simulink model "VehicleControl"  (R2021b)
settings: Solver=FixedStepDiscrete  StartTime=0.0  StopTime=10.0  FixedStep=0.01  RelTol=1e-3
undefined symbols (not defined in the file): DiscIntNeverNeededParam
libraries: simulink x9, simulink_extras x1
settings Model: Creator=Admin  LastModifiedBy=Admin
settings OptimizationCC: DefaultParameterBehavior=Inlined  UseDivisionForNetSlopeComputation=on  GainParamInheritBuiltInType=on  UseFloatMulNetSlope=on  InlineInvariantSignals=on  PassReuseOutputArgsAs=Individual arguments  ZeroExternalMemoryAtStartup=off  ZeroInternalMemoryAtStartup=off  NoFixptDivByZeroProtection=on  EfficientFloat2IntCast=on  LifeSpan=1  OptimizeBlockOrder=speed  DifferentSizesBufferReuse=on  EfficientTunableParamExpr=on
settings DebuggingCC: ParameterTunabilityLossMsg=error
settings HardwareCC: ProdLongLongMode=on
settings ModelReferenceCC: EnableRefExpFcnMdlSchedulingChecks=off
settings SFSimCC: MATLABDynamicMemAlloc=off
settings RTWCC: Description=Embedded Coder  SystemTargetFile=ert.tlc  PackageName=RemoteControllerCodeGen  TemplateMakefile=ert_default_tmf
settings CodeAppCC: ForceParamTrailComments=on  IgnoreCustomStorageClasses=off  OperatorAnnotations=on  SimulinkDataObjDesc=on  SFDataObjDesc=on  CustomSymbolStrGlobalVar=rt$N$M  CustomSymbolStrType=$N$M  CustomSymbolStrFcn=$N$M$F  CustomSymbolStrMacro=$N$M  InsertBlockDesc=on
settings ERTTargetCC: TargetLangStandard=C99 (ISO)  GenerateSampleERTMain=on  IncludeMdlTerminateFcn=off  CombineSignalStateStructs=on  SupportAbsoluteTime=off  SupportComplex=off  SupportNonInlinedSFcns=on  InlinedParameterPlacement=NonHierarchical  ERTCustomFileTemplate=example_file_process.tlc  ERTFilePackagingFormat=CompactWithDataFile

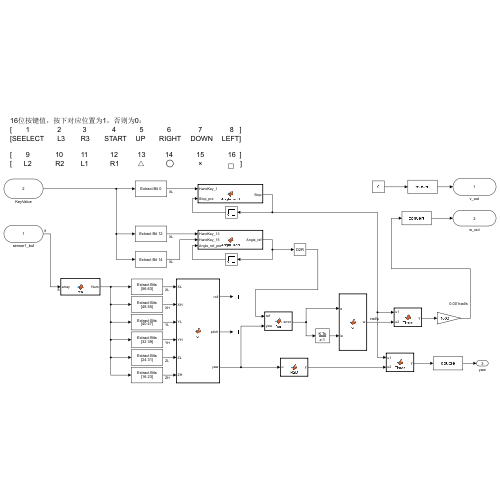
[thumbnail: Simulink's stored preview of the top-level diagram]
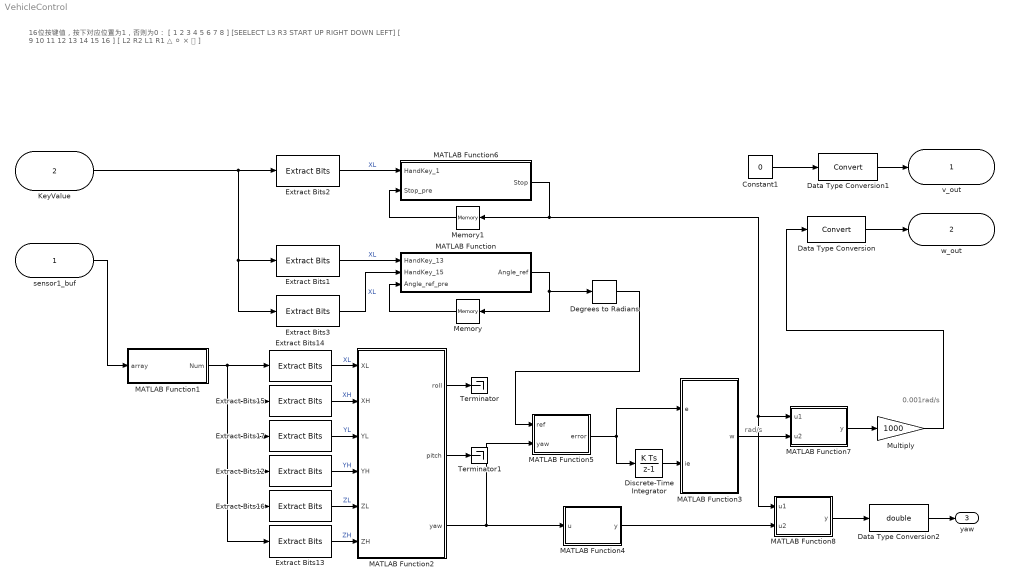
== system VehicleControl ==
  note: 16位按键值，按下对应位置为1，否则为0：
      | [ 1 2 3 4 5 6 7 8 ]
      | [SEELECT L3 R3 START UP RIGHT DOWN LEFT]
      |
      | [ 9 10 11 12 13 14 15 16 ]
      | [ L2 R2 L1 R1 △ ⚪ × ⃞ ]
  note: 0.001rad/s
  note: rad/s
  sensor1_buf : Inport  OutDataTypeStr=int8  PortDimensions=8
  KeyValue : Inport  Port=2  OutDataTypeStr=uint16  PortDimensions=1
  Constant1 : Constant  Value=0  OutDataTypeStr=uint8  SampleTime=-1
  Data Type Conversion : DataTypeConversion
  Data Type Conversion1 : DataTypeConversion
  Data Type Conversion2 : DataTypeConversion  OutDataTypeStr=double
  Degrees to Radians : simulink_extras/Transformations/Degrees to Radians
  Discrete-Time Integrator : DiscreteIntegrator  SampleTime=-1  ICPrevOutput=DiscIntNeverNeededParam  ICPrevScaledInput=DiscIntNeverNeededParam
  Extract Bits1 : simulink/Logic and Bit Operations/Extract Bits  bitsToExtract=Range of bits  numBits=8  bitIdxRange=[12]  outScalingMode=Treat bit field as an integer
  Extract Bits12 : simulink/Logic and Bit Operations/Extract Bits  bitsToExtract=Range of bits  numBits=8  bitIdxRange=[32 39]  outScalingMode=Treat bit field as an integer
  Extract Bits13 : simulink/Logic and Bit Operations/Extract Bits  bitsToExtract=Range of bits  numBits=8  bitIdxRange=[16 23]  outScalingMode=Treat bit field as an integer
  Extract Bits14 : simulink/Logic and Bit Operations/Extract Bits  bitsToExtract=Range of bits  numBits=8  bitIdxRange=[56 63]  outScalingMode=Treat bit field as an integer
  Extract Bits15 : simulink/Logic and Bit Operations/Extract Bits  bitsToExtract=Range of bits  numBits=8  bitIdxRange=[48 55]  outScalingMode=Treat bit field as an integer
  Extract Bits16 : simulink/Logic and Bit Operations/Extract Bits  bitsToExtract=Range of bits  numBits=8  bitIdxRange=[24 31]  outScalingMode=Treat bit field as an integer
  Extract Bits17 : simulink/Logic and Bit Operations/Extract Bits  bitsToExtract=Range of bits  numBits=8  bitIdxRange=[40 47]  outScalingMode=Treat bit field as an integer
  Extract Bits2 : simulink/Logic and Bit Operations/Extract Bits  bitsToExtract=Range of bits  numBits=8  bitIdxRange=[0]  outScalingMode=Treat bit field as an integer
  Extract Bits3 : simulink/Logic and Bit Operations/Extract Bits  bitsToExtract=Range of bits  numBits=8  bitIdxRange=[14]  outScalingMode=Treat bit field as an integer
  MATLAB Function : MATLAB Function  TreatAsAtomicUnit=on
  MATLAB Function1 : MATLAB Function  TreatAsAtomicUnit=on
  MATLAB Function2 : MATLAB Function  TreatAsAtomicUnit=on
  MATLAB Function3 : MATLAB Function  TreatAsAtomicUnit=on
  MATLAB Function4 : MATLAB Function  TreatAsAtomicUnit=on
  MATLAB Function5 : MATLAB Function  TreatAsAtomicUnit=on
  MATLAB Function6 : MATLAB Function  TreatAsAtomicUnit=on
  MATLAB Function7 : MATLAB Function  TreatAsAtomicUnit=on
  MATLAB Function8 : MATLAB Function  TreatAsAtomicUnit=on
  Memory : Memory
  Memory1 : Memory
  Multiply : Gain  Gain=1000  OutDataTypeStr=double
  Terminator : Terminator
  Terminator1 : Terminator
  v_out : Outport  OutDataTypeStr=double
  w_out : Outport  Port=2  OutDataTypeStr=double
  yaw : Outport  Port=3  OutDataTypeStr=double
  wires:
  Extract Bits14/1 -> MATLAB Function2/1(XL)  "XL"
  Extract Bits15/1 -> MATLAB Function2/2(XH)  "XH"
  Extract Bits17/1 -> MATLAB Function2/3(YL)  "YL"
  Extract Bits13/1 -> MATLAB Function2/6(ZH)  "ZH"
  Extract Bits12/1 -> MATLAB Function2/4(YH)  "YH"
  Extract Bits16/1 -> MATLAB Function2/5(ZL)  "ZL"
  MATLAB Function1/1(Num) -> Extract Bits13/1, Extract Bits16/1, Extract Bits12/1, Extract Bits17/1, Extract Bits15/1, Extract Bits14/1
  MATLAB Function5/1(error) -> MATLAB Function3/1(e), Discrete-Time Integrator/1
  Constant1/1 -> Data Type Conversion1/1
  Multiply/1 -> Data Type Conversion/1
  Data Type Conversion/1 -> w_out/1
  Data Type Conversion1/1 -> v_out/1
  Data Type Conversion2/1 -> yaw/1
  MATLAB Function2/2(pitch) -> Terminator1/1
  MATLAB Function2/1(roll) -> Terminator/1
  MATLAB Function2/3(yaw) -> MATLAB Function5/2(yaw), MATLAB Function4/1(u)
  sensor1_buf/1 -> MATLAB Function1/1(array)
  Discrete-Time Integrator/1 -> MATLAB Function3/2(ie)
  KeyValue/1 -> Extract Bits3/1, Extract Bits1/1, Extract Bits2/1
  Extract Bits1/1 -> MATLAB Function/1(HandKey_13)  "XL"
  MATLAB Function/1(Angle_ref) -> Memory/1, Degrees to Radians/1
  Memory/1 -> MATLAB Function/3(Angle_ref_pre)
  Extract Bits2/1 -> MATLAB Function6/1(HandKey_1)  "XL"
  Memory1/1 -> MATLAB Function6/2(Stop_pre)
  MATLAB Function3/1(w) -> MATLAB Function7/2(u2)
  MATLAB Function7/1(y) -> Multiply/1
  MATLAB Function4/1(y) -> MATLAB Function8/2(u2)
  MATLAB Function8/1(y) -> Data Type Conversion2/1
  MATLAB Function6/1(Stop) -> MATLAB Function8/1(u1), MATLAB Function7/1(u1), Memory1/1
  Degrees to Radians/1 -> MATLAB Function5/1(ref)
  Extract Bits3/1 -> MATLAB Function/2(HandKey_15)  "XL"

== matlab function VehicleControl/MATLAB Function1 ==
  data: array input; Num output
function Num = fcn(array)
Num=int64(0);
len = length(array);
    for i=1:len
            Num = bitshift(Num,8)+int64(array(i));
    end
Num = int64(Num);
end

== matlab function VehicleControl/MATLAB Function ==
  data: HandKey_13 input; HandKey_15 input; Angle_ref output; Angle_ref_pre input
function Angle_ref = Angle_add(HandKey_13,HandKey_15,Angle_ref_pre)

Angle_ref = 0;

if HandKey_13 == 0
    Angle_ref = Angle_ref_pre + 3;
    if Angle_ref >= 350
        Angle_ref = 350;
    end
elseif HandKey_15 == 0
    Angle_ref = Angle_ref_pre - 3;
    if Angle_ref <= 10
        Angle_ref = 10;
    end
else
    Angle_ref = Angle_ref_pre;
end

== matlab function VehicleControl/MATLAB Function3 ==
  data: w output; e input; ie input
function w  = fcn(e,ie)

Kp = 1.2;
Ki = 0;
w = -Kp*e-Ki*ie;

== matlab function VehicleControl/MATLAB Function4 ==
  data: u input; y output
function y = R2D(u)

y = double(u)/pi*180;

== matlab function VehicleControl/MATLAB Function5 ==
  data: ref input; error output; yaw input
function error = fcn(ref,yaw)

error = -yaw+ref;

== matlab function VehicleControl/MATLAB Function6 ==
  data: HandKey_1 input; Stop output; Stop_pre input
function Stop = Angle_add(HandKey_1,Stop_pre)

Stop = 0;
Stop = Stop_pre;
if HandKey_1 == 0
    if Stop_pre == 0
        Stop = 1;
    else
        Stop = 0;
    end
end

== matlab function VehicleControl/MATLAB Function7 ==
  data: u1 input; y output; u2 input
function y = Times(u1,u2)

y = u1*u2;

== matlab function VehicleControl/MATLAB Function8 ==
  data: u1 input; y output; u2 input
function y = Times(u1,u2)

y = u1*u2;

== matlab function VehicleControl/MATLAB Function2 ==
  data: roll output; pitch output; yaw output; XL input; XH input; YL input; YH input; ZL input; ZH input
function [roll,pitch,yaw] = fcn(XL,XH,YL,YH,ZL,ZH)
XL = int16(XL);
XH = int16(XH);
YL = int16(YL);
YH = int16(YH);
ZL = int16(ZL);
ZH = int16(ZH);
a=bitshift(XH,8)+XL;
b=bitshift(YH,8)+YL;
c=int16(bitshift(ZH,8))+int16(ZL);
roll=double(a)*pi/(100*180);
pitch=double(b)*pi/(100*180);
yaw=double(c)*pi/(100*180);
